simulink model "LIN_VEL_usporedba"  (R2020b)
settings: Solver=VariableStepAuto  StartTime=0.0  StopTime=10.0  RelTol=1e-3
undefined symbols (not defined in the file): k_z, wn_z
settings Model: Creator=Ivan  LastModifiedBy=Ivan

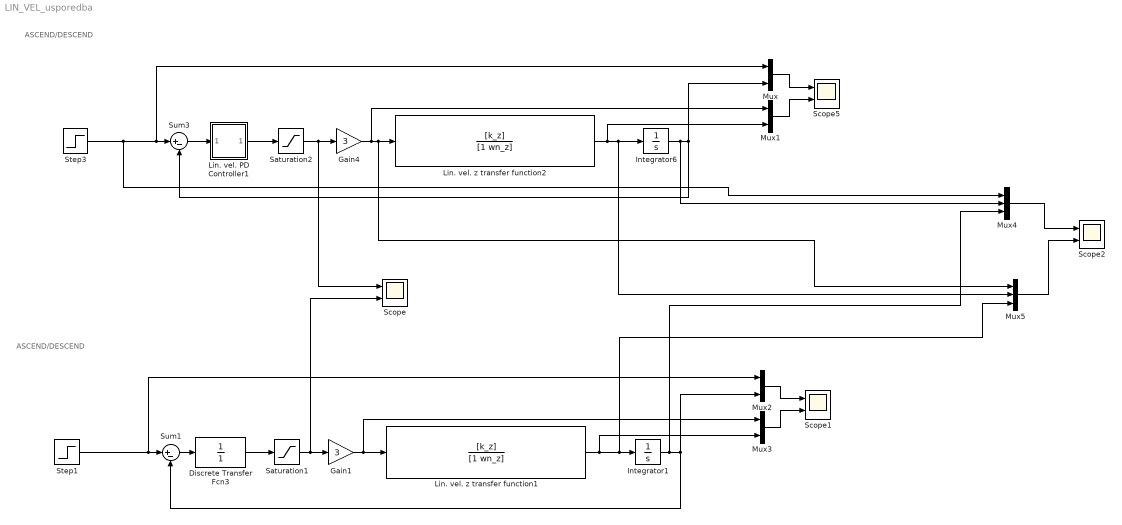
== system LIN_VEL_usporedba ==
  note: ASCEND/DESCEND
  note: ASCEND/DESCEND
  Discrete Transfer Fcn3 : DiscreteTransferFcn  Denominator=[1]  SampleTime=0.1
  Gain1 : Gain  Gain=3
  Gain4 : Gain  Gain=3
  Integrator1 : Integrator
  Integrator6 : Integrator
  Lin. vel. PD Controller1 : Subsystem
  Lin. vel. z transfer function1 : TransferFcn  Numerator=[k_z]  Denominator=[1 wn_z]
  Lin. vel. z transfer function2 : TransferFcn  Numerator=[k_z]  Denominator=[1 wn_z]
  Mux{,1..3} (4 alike) : Mux  Inputs=2
  Mux4 : Mux  Inputs=3
  Mux5 : Mux  Inputs=3
  Saturation1 : Saturate  UpperLimit=1  LowerLimit=-1
  Saturation2 : Saturate  UpperLimit=1  LowerLimit=-1
  Scope{,1..2,5} (4 alike) : Scope  NumInputPorts=2
  Step1 : Step  Time=0  SampleTime=0
  Step3 : Step  Time=0  SampleTime=0
  Sum1 : Sum  Inputs=|+-
  Sum3 : Sum  Inputs=|+-
  wires:
  Mux1/1 -> Scope5/2
  Sum3/1 -> Lin. vel. PD Controller1/1("  ")
  Lin. vel. PD Controller1/1(" ") -> Saturation2/1
  Saturation2/1 -> Scope/1, Gain4/1
  Mux/1 -> Scope5/1
  Integrator6/1 -> Mux4/2, Mux/2, Sum3/2
  Step3/1 -> Mux4/1, Mux/1, Sum3/1
  Gain4/1 -> Mux1/1, Mux5/1, Lin. vel. z transfer function2/1
  Lin. vel. z transfer function2/1 -> Mux1/2, Mux5/2, Integrator6/1
  Discrete Transfer Fcn3/1 -> Saturation1/1
  Mux2/1 -> Scope1/1
  Sum1/1 -> Discrete Transfer Fcn3/1
  Mux3/1 -> Scope1/2
  Saturation1/1 -> Scope/2, Gain1/1
  Lin. vel. z transfer function1/1 -> Mux3/2, Mux5/3, Integrator1/1
  Integrator1/1 -> Mux4/3, Mux2/2, Sum1/2
  Gain1/1 -> Mux3/1, Lin. vel. z transfer function1/1
  Step1/1 -> Mux2/1, Sum1/1
  Mux5/1 -> Scope2/2
  Mux4/1 -> Scope2/1

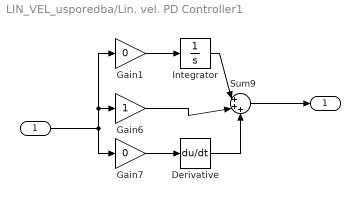
== system LIN_VEL_usporedba/Lin. vel. PD Controller1 ==
  "  " : Inport
  Derivative : Derivative
  Gain1 : Gain  Gain=0
  Gain6 : Gain
  Gain7 : Gain  Gain=0
  Integrator : Integrator
  Sum9 : Sum  Inputs=|+++
  " " : Outport
  wires:
  Sum9/1 -> " "/1
  Gain7/1 -> Derivative/1
  Gain6/1 -> Sum9/2
  Derivative/1 -> Sum9/3
  "  "/1 -> Gain1/1, Gain6/1, Gain7/1
  Integrator/1 -> Sum9/1
  Gain1/1 -> Integrator/1
